simulink model "MPSLab1Igor"  (R2014b)
settings: Solver=ode45  StartTime=0.0  StopTime=50  RelTol=1e-3
undefined symbols (not defined in the file): magnitude
settings Model: Creator=kiril_000  LastModifiedBy=kiril_000

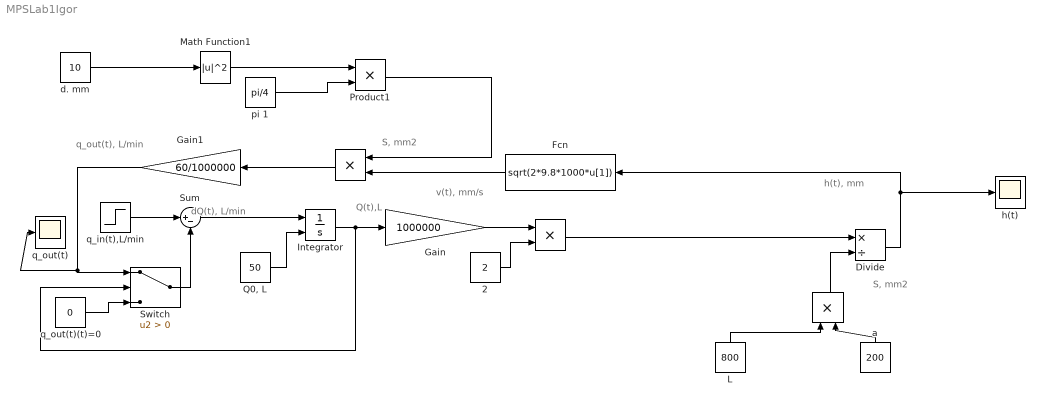
== system MPSLab1Igor ==
  note: h(t), mm
  note: S, mm2
  note: v(t), mm/s
  note: q_out(t), L/min
  note: S, mm2
  note: Q(t),L
  note: dQ(t), L/min
  " " : Product
  "  " : Product
  "   " : Product
  2 : Constant  Value=2
  Divide : Product  Inputs=*/
  Fcn : Fcn  Expr=sqrt(2*9.8*1000*u[1])
  Gain : Gain  Gain=1000000
  Gain1 : Gain  Gain=60/1000000
  Integrator : Integrator  InitialConditionSource=external
  L : Constant  Value=800
  Math Function1 : Math  Operator=magnitude^2  SaturateOnIntegerOverflow=on
  Product1 : Product
  "Q0, L" : Constant  Value=50
  Sum : Sum  Inputs=|+-
  Switch : Switch  Criteria=u2 > Threshold
  a : Constant  Value=200
  d. mm : Constant  Value=10
  h(t) : Scope
      settings: TimeRange=30  YMin=-100  YMax=600
  pi 1 : Constant  Value=pi/4
  q_in(t),L/min : Step  Time=10  After=12  SampleTime=0
  q_out(t) : Scope
  q_out(t)(t)=0 : Constant  Value=0
  wires:
  q_in(t),L/min/1 -> Sum/1
  q_out(t)(t)=0/1 -> Switch/3
  Sum/1 -> Integrator/1
  "Q0, L"/1 -> Integrator/2
  Switch/1 -> Sum/2
  Integrator/1 -> Switch/2, Gain/1
  Divide/1 -> Fcn/1, h(t)/1
  d. mm/1 -> Math Function1/1
  Math Function1/1 -> Product1/1
  pi 1/1 -> Product1/2
  Product1/1 -> "   "/1
  "   "/1 -> Gain1/1
  Fcn/1 -> "   "/2
  2/1 -> " "/2
  Gain/1 -> " "/1
  " "/1 -> Divide/1
  "  "/1 -> Divide/2
  Gain1/1 -> Switch/1, q_out(t)/1
  a/1 -> "  "/2
  L/1 -> "  "/1
